simulink model "Decuplarea"  (R2018a)
settings: Solver=VariableStepAuto  StartTime=0.0  StopTime=100  RelTol=1e-3
undefined symbols (not defined in the file or in its folder): dem11, dem12, dem21, dem22, demcon11, demcon22, demD12, demD21, demgg11, demgg12, demgg21, demgg22, demh11, demh12, demh21, demh22, num11, num12, num21, num22, numcon11, numcon22, numD12, numD21, numgg11, numgg12, numgg21, numgg22, numh11, numh12, numh21, numh22
settings Model: Creator=Andrei  LastModifiedBy=Andrei

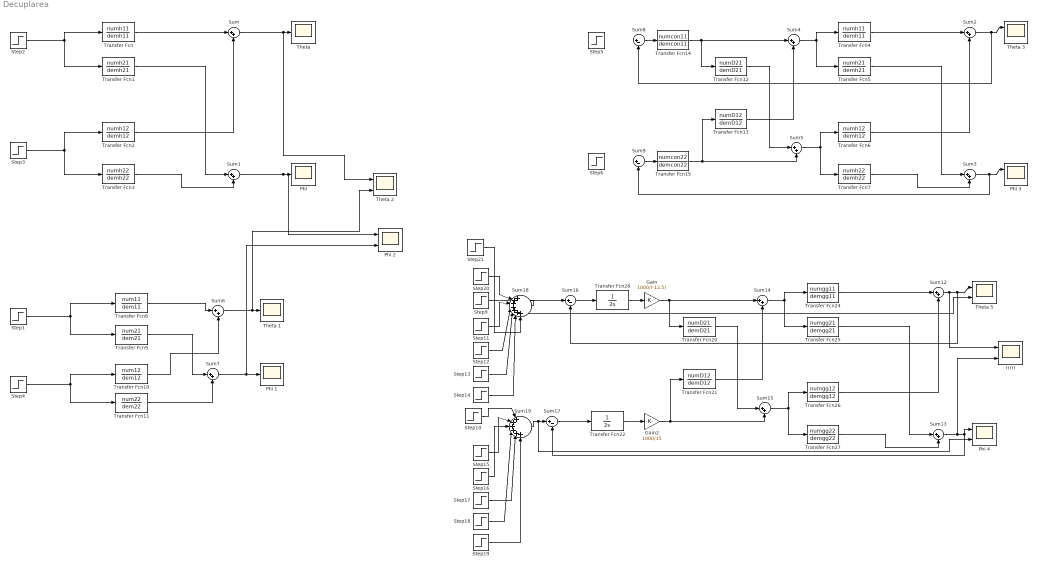
== system Decuplarea ==
  Gain : Gain  Gain=1000/(-12.5)
  Gain2 : Gain  Gain=1000/15
  "Phi " : Scope
  Phi 1 : Scope
  Phi 2 : Scope  NumInputPorts=2
  Phi 3 : Scope  NumInputPorts=2
  Phi 4 : Scope  NumInputPorts=2
  Step{1..5,20} (6 alike) : Step  Time=0  SampleTime=0
  Step10 : Step  Time=0  After=4  SampleTime=0
  Step11 : Step  Time=30  After=14  SampleTime=0
  Step12 : Step  Time=45  After=-38  SampleTime=0
  Step13 : Step  Time=60  After=77  SampleTime=0
  Step14 : Step  Time=75  After=-100  SampleTime=0
  Step15 : Step  Time=10  After=-20  SampleTime=0
  Step16 : Step  Time=20  After=-75  SampleTime=0
  Step17 : Step  Time=40  After=50  SampleTime=0
  Step18 : Step  Time=60  After=-100  SampleTime=0
  Step19 : Step  Time=85  After=140  SampleTime=0
  Step21 : Step  Time=90  After=25  SampleTime=0
  Step6 : Step  Time=0.5  After=10  SampleTime=0
  Step9 : Step  Time=15  After=-6  SampleTime=0
  Sum{,1..7,12..15} (12 alike) : Sum  Inputs=|++
  Sum{8..9,16..17} (4 alike) : Sum  Inputs=|+-
  Sum18 : Sum  Inputs=|+++++++
  Sum19 : Sum  Inputs=|++++++
  "Theta " : Scope
  Theta 1 : Scope
  Theta 2 : Scope  NumInputPorts=2
  Theta 3 : Scope  NumInputPorts=2
  Theta 5 : Scope  NumInputPorts=2
  Transfer Fcn : TransferFcn  Numerator=numh11  Denominator=demh11
  Transfer Fcn1 : TransferFcn  Numerator=numh21  Denominator=demh21
  Transfer Fcn10 : TransferFcn  Numerator=num12  Denominator=dem12
  Transfer Fcn11 : TransferFcn  Numerator=num22  Denominator=dem22
  Transfer Fcn12 : TransferFcn  Numerator=numD21  Denominator=demD21
  Transfer Fcn13 : TransferFcn  Numerator=numD12  Denominator=demD12
  Transfer Fcn14 : TransferFcn  Numerator=numcon11  Denominator=demcon11
  Transfer Fcn15 : TransferFcn  Numerator=numcon22  Denominator=demcon22
  Transfer Fcn2 : TransferFcn  Numerator=numh12  Denominator=demh12
  Transfer Fcn20 : TransferFcn  Numerator=numD21  Denominator=demD21
  Transfer Fcn21 : TransferFcn  Numerator=numD12  Denominator=demD12
  Transfer Fcn22 : TransferFcn  Denominator=[2 0]
  Transfer Fcn24 : TransferFcn  Numerator=numgg11  Denominator=demgg11
  Transfer Fcn25 : TransferFcn  Numerator=numgg21  Denominator=demgg21
  Transfer Fcn26 : TransferFcn  Numerator=numgg12  Denominator=demgg12
  Transfer Fcn27 : TransferFcn  Numerator=numgg22  Denominator=demgg22
  Transfer Fcn28 : TransferFcn  Denominator=[2 0]
  Transfer Fcn3 : TransferFcn  Numerator=numh22  Denominator=demh22
  Transfer Fcn4 : TransferFcn  Numerator=numh11  Denominator=demh11
  Transfer Fcn5 : TransferFcn  Numerator=numh21  Denominator=demh21
  Transfer Fcn6 : TransferFcn  Numerator=numh12  Denominator=demh12
  Transfer Fcn7 : TransferFcn  Numerator=numh22  Denominator=demh22
  Transfer Fcn8 : TransferFcn  Numerator=num11  Denominator=dem11
  Transfer Fcn9 : TransferFcn  Numerator=num21  Denominator=dem21
  "rrrrr " : Scope  NumInputPorts=2
  wires:
  Sum1/1 -> Phi 2/1, "Phi "/1
  Transfer Fcn/1 -> Sum/1
  Sum/1 -> Theta 2/1, "Theta "/1
  Transfer Fcn2/1 -> Sum/2
  Transfer Fcn3/1 -> Sum1/2
  Step4/1 -> Transfer Fcn11/1, Transfer Fcn10/1
  Step1/1 -> Transfer Fcn9/1, Transfer Fcn8/1
  Transfer Fcn8/1 -> Sum6/1
  Transfer Fcn9/1 -> Sum7/1
  Sum6/1 -> Theta 2/2, Theta 1/1
  Sum7/1 -> Phi 2/2, Phi 1/1
  Transfer Fcn10/1 -> Sum6/2
  Transfer Fcn11/1 -> Sum7/2
  Step2/1 -> Transfer Fcn1/1, Transfer Fcn/1
  Step3/1 -> Transfer Fcn3/1, Transfer Fcn2/1
  Transfer Fcn1/1 -> Sum1/1
  Transfer Fcn7/1 -> Sum3/2
  Transfer Fcn6/1 -> Sum2/2
  Transfer Fcn5/1 -> Sum3/1
  Transfer Fcn4/1 -> Sum2/1
  Sum2/1 -> Sum8/2, Theta 3/1
  Sum3/1 -> Sum9/2, Phi 3/1
  Sum4/1 -> Transfer Fcn5/1, Transfer Fcn4/1
  Sum5/1 -> Transfer Fcn6/1, Transfer Fcn7/1
  Sum8/1 -> Transfer Fcn14/1
  Sum9/1 -> Transfer Fcn15/1
  Transfer Fcn13/1 -> Sum4/2
  Transfer Fcn12/1 -> Sum5/1
  Transfer Fcn14/1 -> Sum4/1, Transfer Fcn12/1
  Transfer Fcn15/1 -> Transfer Fcn13/1, Sum5/2
  Transfer Fcn21/1 -> Sum14/2
  Sum14/1 -> Transfer Fcn25/1, Transfer Fcn24/1
  Transfer Fcn26/1 -> Sum12/2
  Sum15/1 -> Transfer Fcn26/1, Transfer Fcn27/1
  Sum12/1 -> "rrrrr "/1, Sum16/2, Theta 5/1
  Transfer Fcn27/1 -> Sum13/2
  Transfer Fcn20/1 -> Sum15/1
  Transfer Fcn24/1 -> Sum12/1
  Transfer Fcn25/1 -> Sum13/1
  Gain/1 -> Sum14/1, Transfer Fcn20/1
  Sum13/1 -> "rrrrr "/2, Sum17/2, Phi 4/1
  Gain2/1 -> Transfer Fcn21/1, Sum15/2
  Sum16/1 -> Transfer Fcn28/1
  Sum17/1 -> Transfer Fcn22/1
  Transfer Fcn28/1 -> Gain/1
  Transfer Fcn22/1 -> Gain2/1
  Sum18/1 -> Theta 5/2, Sum16/1
  Step9/1 -> Sum18/1
  Step10/1 -> Sum19/1
  Sum19/1 -> Phi 4/2, Sum17/1
  Step11/1 -> Sum18/3
  Step12/1 -> Sum18/4
  Step13/1 -> Sum18/5
  Step14/1 -> Sum18/6
  Step15/1 -> Sum19/2
  Step16/1 -> Sum19/3
  Step20/1 -> Sum18/2
  Step18/1 -> Sum19/4
  Step17/1 -> Sum19/5
  Step19/1 -> Sum19/6
  Step21/1 -> Sum18/7
